simulink model "inv_pend_losses"  (Simulink 7.6)
settings: Solver=ode45  StartTime=0.0  StopTime=2  RelTol=1e-3
libraries: simulink x1
settings Model: Creator=mengg_000  LastModifiedBy=mengg
settings DebuggingCC: InheritedTsInSrcMsg=none

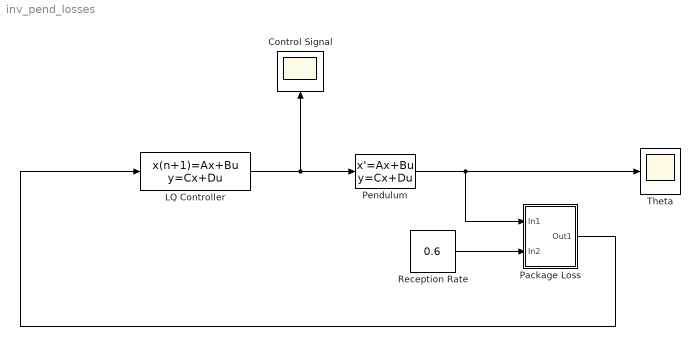
== system inv_pend_losses ==
  Control Signal : Scope
      settings: TimeRange=1  YMin=1  YMax=3.5  SaveName=ry
  LQ Controller : DiscreteStateSpace  A=|  B=|  C="[-12.1798  -13.3262         0]"  D=-8.1263  X0="[0;    0;   0]"  SampleTime=0.02
      A=|
      | [0.0389   -1.5001         0;
      |     0.0828    0.3594         0;
      |   -12.1798  -13.3262         0]
      B=|
      | [ -0.4344;
      |     0.1355;
      |    -8.1263]
  Package Loss : Subsystem
  "Pendulum " : StateSpace  A=[0 3.0628;32 0]  B=[2; 0]  C=[0 1.5314]  D=0  X0=[0; 0.1]
  Reception Rate : Constant  Value=0.6
  Theta : Scope
      settings: TimeRange=1  YMin=1  YMax=3.5  SaveName=ry1
  wires:
  "Pendulum "/1 -> Theta/1, Package Loss/1(In1)
  LQ Controller/1 -> "Pendulum "/1, Control Signal/1
  Reception Rate/1 -> Package Loss/2(In2)
  Package Loss/1(Out1) -> LQ Controller/1

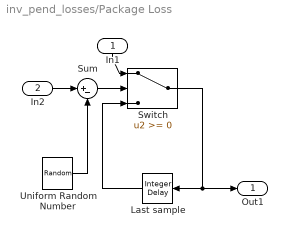
== system inv_pend_losses/Package Loss ==
  In1 : Inport
  In2 : Inport  Port=2
  Last sample : simulink/Discrete/Integer Delay  NumDelays=1  vinit=0.0  samptime=-1
  Sum : Sum  Inputs=|+-
  Switch : Switch
  Uniform Random Number : UniformRandomNumber  Minimum=0
  Out1 : Outport
  wires:
  Uniform Random Number/1 -> Sum/2
  Sum/1 -> Switch/2
  In1/1 -> Switch/1
  In2/1 -> Sum/1
  Switch/1 -> Out1/1, Last sample/1
  Last sample/1 -> Switch/3
